simulink model "ForSerial"  (R2018b)
settings: Solver=ode4  StartTime=0.0  StopTime=20.0  FixedStep=1e-3  RelTol=1e-3
undefined symbols (not defined in the file): serial
libraries: instrumentlib x2
settings Model: Creator=shnuer  LastModifiedBy=shnuer
settings DataIOCC: SaveFormat=StructureWithTime

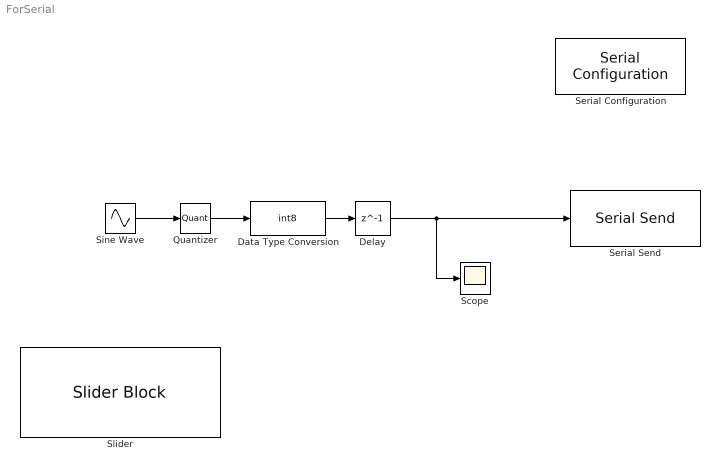
== system ForSerial ==
  Data Type Conversion : DataTypeConversion  OutDataTypeStr=int8
  Delay : Delay  DelayLength=1  InitialCondition=0
  Quantizer : Quantizer  QuantizationInterval=1
  Scope : Scope
  Serial Configuration : instrumentlib/Serial Configuration  Priority=-200000  ComPortMenu=/dev/ttyUSB0  ComPort=/dev/ttyUSB0  ObjConstructor=serial('/dev/ttyUSB0');  BaudRate=115200  DataBits=8  Parity=none  StopBits=1  FlowControl=none  Timeout=10  ByteOrder=LittleEndian
  Serial Send : instrumentlib/Serial Send  ComPortMenu=<Please select a port...>  ComPort=/dev/ttyUSB0  ObjConstructor=serial('/dev/ttyUSB0');  Terminator=<none>  EnableBlockingMode=on
  Sine Wave : Sin  Bias=1  SampleTime=1
  Slider : SliderBlock  WebBlockId=24  LabelPosition=Bottom  ScaleMin=1  ScaleMax=3  TickInterval=1
  wires:
  Data Type Conversion/1 -> Delay/1
  Delay/1 -> Scope/1, Serial Send/1
  Quantizer/1 -> Data Type Conversion/1
  Sine Wave/1 -> Quantizer/1
